simulink model "VTOL_sim"  (R2016b)
settings: Solver=ode45  StartTime=0.0  StopTime=10000  RelTol=1e-3  EnableMultiTasking=on
InitFcn:
  | addpath ./..
  | VTOL_param
undefined symbols (not defined in the file): P, VTOL_animation
libraries: simulink x4
settings Model: Creator=beard  LastModifiedBy=beard
settings DataIOCC: LimitDataPoints=on  SaveFormat=Array  SignalLoggingSaveFormat=ModelDataLogs
settings OptimizationCC: ExpressionDepthLimit=2147483647  InitFltsAndDblsToZero=on  LifeSpan=inf
settings DebuggingCC: UnderspecifiedInitializationDetection=Classic  MergeDetectMultiDrivingBlocksExec=none  SolverPrmCheckMsg=warning  FcnCallInpInsideContextMsg=warning  StateNameClashWarn=warning  SFUnexpectedBacktrackingDiag=warning  SFNoUnconditionalDefaultTransitionDiag=warning  SFExecutionAtInitializationDiag=none
settings HardwareCC: ProdBitPerPointer=32  ProdBitPerSizeT=32  ProdBitPerPtrDiffT=32  ProdLargestAtomicFloat=None  ProdIntDivRoundTo=Undefined  ProdEndianess=Unspecified  ProdWordSize=32  ProdHWDeviceType=32-bit Generic
settings ModelReferenceCC: PropagateSignalLabelsOutOfModel=off
settings GRTTargetCC: TargetLangStandard=C89/C90 (ANSI)  GeneratePreprocessorConditionals=Disable all  CombineOutputUpdateFcns=off  GRTInterface=on
settings ConfigComp: CovMetricSettings=dw  CovHtmlReporting=on  CovSaveCumulativeToWorkspaceVar=on  CovSaveSingleToWorkspaceVar=on  CovExternalEMLEnable=off

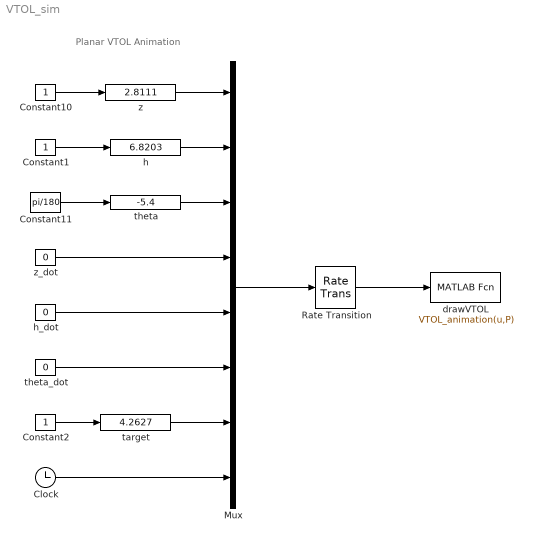
== system VTOL_sim ==
  note: Planar VTOL Animation
  Clock : Clock
  Constant1 : Constant
  Constant10 : Constant
  Constant11 : Constant  Value=pi/180
  Constant2 : Constant
  Mux : Mux  Inputs=8
  Rate Transition : RateTransition  OutPortSampleTime=P.t_plot
  drawVTOL : MATLABFcn  MATLABFcn=VTOL_animation(u,P)  OutputDimensions=0
  h : simulink/Math Operations/Slider Gain  low=0  gain=6.8203  high=10
  h_dot : Constant  Value=0
  target : simulink/Math Operations/Slider Gain  low=0  gain=4.2627  high=5
  theta : simulink/Math Operations/Slider Gain  low=-90  gain=-5.4  high=90
  theta_dot : Constant  Value=0
  z : simulink/Math Operations/Slider Gain  low=0  gain=2.8111  high=10
  "z_dot " : Constant  Value=0
  wires:
  z/1 -> Mux/1
  Constant10/1 -> z/1
  theta/1 -> Mux/3
  Constant11/1 -> theta/1
  Mux/1 -> Rate Transition/1
  Constant1/1 -> h/1
  h/1 -> Mux/2
  Constant2/1 -> target/1
  target/1 -> Mux/7
  Clock/1 -> Mux/8
  Rate Transition/1 -> drawVTOL/1
  "z_dot "/1 -> Mux/4
  h_dot/1 -> Mux/5
  theta_dot/1 -> Mux/6
